simulink model "lab5_EAs"  (R2021b)
settings: Solver=VariableStepAuto  StartTime=0.0  StopTime=10.0  RelTol=1e-3
values from neighbouring files (symbols this model uses):
  J = [Ixx 0 0; 0 Iyy 0; 0 0 Izz]    [lab5_task1.m]
  Jinv = inv(J)    [lab5_task1.m]
  phi0 = 0    [lab5_task1.m]
  psi0 = 0    [lab5_task1.m]
  theta0 = 0    [lab5_task1.m]
  w0 = [0.45 0.52 0.55]'    [lab5_task1.m]
libraries: matrix_library x1
settings Model: Creator=samuz  LastModifiedBy=samuz

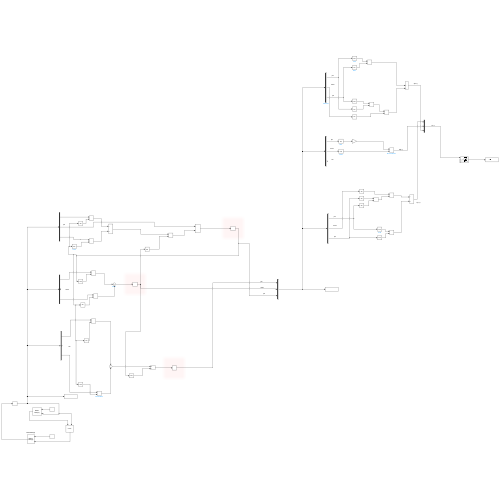
[thumbnail: Simulink's stored preview of the top-level diagram]
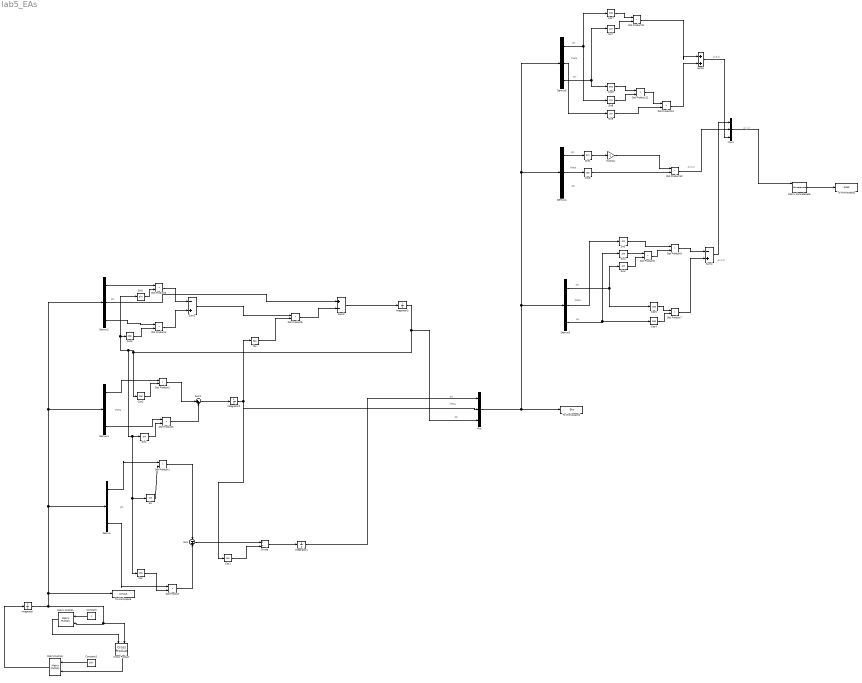
== system lab5_EAs ==
  note: A(:,1)
  note: A(3,1)
  note: A(2,1)
  note: A(1,1)
  note: psi
  note: psi
  note: theta
  note: phi
  note: psi
  note: theta
  note: phi
  note: psi
  note: theta
  note: phi
  note: phi
  note: theta
  note: psi
  note: phi
  note: theta
  Constant : Constant  Value=J
  Constant1 : Constant  Value=Jinv
  Cos{,1..8} (9 alike) : Trigonometry  Operator=cos
  Cross Product : matrix_library/Cross Product
      settings: SourceProductBaseCode=SL
  Demux{,1..5} (6 alike) : Demux  Outputs=3
  Divide : Product  Inputs=*/
  Dot Product{,1..13} (14 alike) : DotProduct  InputSameDT=on  OutDataTypeStr=Inherit: Inherit via internal rule
  Integrator : Integrator  InitialCondition=w0
  Integrator1 : Integrator  InitialCondition=phi0
  Integrator2 : Integrator  InitialCondition=theta0
  Integrator3 : Integrator  InitialCondition=psi0
  Matrix Concatenate : Concatenate  NumInputs=3  Mode=Multidimensional array  ConcatenateDimension=2
  Matrix Multiply : Product  Multiplication=Matrix(*)
  MatrixMultiply : Product  Multiplication=Matrix(*)
  Multiply : Gain  Gain=-1
  Mux : Mux  Inputs=3
  Mux1 : Mux  Inputs=3
  Sin{,1..9} (10 alike) : Trigonometry
  Sum : Sum  Inputs=-+
  Sum1 : Sum  Inputs=|++
  Sum2 : Sum  Inputs=-+
  Sum3 : Sum  Inputs=+-
  Sum4 : Sum  Inputs=-+
  Sum5 : Sum  Inputs=|++
  Tan : Trigonometry  Operator=tan
  To Workspace : ToWorkspace  VariableName=simout  SampleTime=-1
  To Workspace1 : ToWorkspace  VariableName=EAs  SampleTime=-1
  To Workspace2 : ToWorkspace  VariableName=A312  SaveFormat=Timeseries  SampleTime=-1
  wires:
  Cross Product/1 -> MatrixMultiply/2
  Matrix Multiply/1 -> Cross Product/1
  Integrator/1 -> To Workspace/1, Demux2/1, Demux1/1, Demux/1, Cross Product/2, Matrix Multiply/2
  MatrixMultiply/1 -> Integrator/1
  Constant1/1 -> MatrixMultiply/1
  Constant/1 -> Matrix Multiply/1
  Demux/3 -> Dot Product/1
  Cos/1 -> Dot Product/2
  Demux/1 -> Dot Product1/1
  Sin/1 -> Dot Product1/2
  Dot Product1/1 -> Sum/1
  Dot Product/1 -> Sum/2
  Sum/1 -> Divide/1
  Cos1/1 -> Divide/2
  Divide/1 -> Integrator1/1
  Cos2/1 -> Dot Product2/2
  Sin1/1 -> Dot Product3/2
  Demux1/1 -> Dot Product2/1
  Demux1/3 -> Dot Product3/1
  Dot Product2/1 -> Sum1/1
  Dot Product3/1 -> Sum1/2
  Sum1/1 -> Integrator2/1
  Demux2/3 -> Dot Product4/1
  Cos3/1 -> Dot Product4/2
  Sin2/1 -> Dot Product5/2
  Demux2/1 -> Dot Product5/1
  Dot Product4/1 -> Sum2/2
  Dot Product5/1 -> Sum2/1
  Integrator2/1 -> Mux/2, Tan/1, Cos1/1
  Sum2/1 -> Dot Product6/1
  Tan/1 -> Dot Product6/2
  Dot Product6/1 -> Sum3/2
  Demux2/2 -> Sum3/1
  Sum3/1 -> Integrator3/1
  Integrator3/1 -> Cos/1, Sin/1, Sin1/1, Sin2/1, Cos3/1, Cos2/1, Mux/3
  Integrator1/1 -> Mux/1
  Mux/1 -> To Workspace1/1, Demux5/1, Demux4/1, Demux3/1
  Demux3/3 -> Sin4/1, Cos4/1
  Demux3/1 -> Sin3/1, Cos5/1
  Cos5/1 -> Dot Product7/1
  Cos4/1 -> Dot Product7/2
  Demux3/2 -> Sin5/1
  Sin3/1 -> Dot Product8/2
  Sin4/1 -> Dot Product8/1
  Sin5/1 -> Dot Product9/1
  Dot Product8/1 -> Dot Product9/2
  Dot Product9/1 -> Sum4/1
  Dot Product7/1 -> Sum4/2
  Sin6/1 -> Multiply/1
  Demux4/2 -> Cos6/1
  Demux4/1 -> Sin6/1
  Cos6/1 -> Dot Product10/2
  Multiply/1 -> Dot Product10/1
  Demux5/3 -> Sin7/1, Cos8/1
  Demux5/1 -> Cos7/1, Sin8/1
  Cos7/1 -> Dot Product11/1
  Sin7/1 -> Dot Product11/2
  Demux5/2 -> Sin9/1
  Cos8/1 -> Dot Product12/1
  Sin8/1 -> Dot Product12/2
  Dot Product12/1 -> Dot Product13/1
  Sin9/1 -> Dot Product13/2
  Dot Product11/1 -> Sum5/1
  Dot Product13/1 -> Sum5/2
  Sum5/1 -> Mux1/3
  Dot Product10/1 -> Mux1/2
  Sum4/1 -> Mux1/1
  Mux1/1 -> Matrix Concatenate/1
  Matrix Concatenate/1 -> To Workspace2/1
